simulink model "rlHouseHeatingSystem"  (R2023a)
settings: Solver=VariableStepAuto  StartTime=0.0  StopTime=inf  FixedStep=1  MaxStep=50  RelTol=1e-3  AbsTol=1e-3
InitFcn:
  | %   Simscape Demo "House Heating System"
  | % max_temp = 23;    % Maximum temperature
  | % min_temp = 18;     % Minimum temperature
  | % Walls
  | % House length = 30 m
  | lenHouse = 30;
  | % House width = 10 m
  | widHouse = 10;
  | % House height = 4 m
  | htHouse = 4;
  | wallArea = 2*lenHouse*htHouse + 2*widHouse*htHouse;
  | LWall = .2;
  | wallVolume = wallArea * LWall;
  | wallDensity = 1920;     % kg/m^3
  | wallMass = wallVolume * wallDensity;
  | c_wall = 835;           % J/kg/K
  | kWall = 0.038;  % Thermal conductivity [W/m/K]
  | % -------------------------------
  | % Windows
  | % Number of windows = 6
  | numWindows = 6;
  | % Height of windows = 1 m
  | htWindows = 1;
  | % Width of windows = 1 m
  | widWindows = 1;
  | windowArea = numWindows*htWindows*widWindows;
  | LWindow = .01;
  | windowVolume = windowArea * LWindow;
  | windowDensity = 2700;       % kg/m^3
  | windowMass = windowVolume * windowDensity;
  | c_window = 840;             % J/kg/K
  | kWindow = 0.78;             % Thermal conductivity [W/m/K]
  | % -------------------------------
  | % Roof
  | % Roof pitch = 40 deg
  | pitRoof = 40/180/pi;
  | roofArea =  2*(1/cos(pitRoof/2))*widHouse*lenHouse + tan(pitRoof)*widHouse;
  | LRoof = 0.2;
  | roofVolume = roofArea * LRoof;
  | roofDensity = 32;           % Glass fiber
  | roofMass = roofVolume * roofDensity;
  | kRoof = 0.038;              % Thermal conductivity [W/m/K]
  | c_roof = 835;               % J/kg/K
  | % -------------------------------
  | % Convective heat gransfer coefficients (W/M^2/K)
  | h_A_W = 24;         % Air-wall
  | h_W_Atm = 34;       % Wall-atmosphere
  | h_A_Wnd = 25;       % Air-window
  | h_Wnd_Atm = 32;     % Window-atmosphere
  | h_A_R = 12;         % Air-roof
  | h_R_Atm = 38;       % Roof-atmosphere
  | % -------------------------------
  | %Air
  | % Density of air at sea level = 1.2250 kg/m^3
  | densAir = 1.2250;
  | % Air mass inside the house
  | M_air = (lenHouse*widHouse*htHouse+tan(pitRoof)*widHouse*lenHouse)*densAir;
  | c_air = 1005.4;         % cp of air at 273 K [J/(kg*K]
  | % -------------------------------
  | % Heater
  | % The air exiting the heater has a constant temperature which is a heater
  | % property. THeater = 50 deg C
  | THeater = 50;
  | HeaterAirFlow = 1;  % Heater air flow rate [kg/s]
  | % -------------------------------
  | % Cost of electricity
  | % Assume the cost of electricity is $0.09 per kilowatt/hour
  | % Assume all electric energy is transformed to heat energy
  | % 1 kW-hr = 3.6e6 J
  | % cost = $0.09 per 3.6e6 J
  | cost = 0.09/3.6e6;
  | % -------------------------------
  | % Initial internal temperatures
  | TinIC = 20; % deg C
values from neighbouring files (symbols this model uses):
  comfortMax = 23    [1_initialhouseheatingmodel.m]
  comfortMin = 18    [1_initialhouseheatingmodel.m]
libraries: fl_lib x22, nesl_utility_internal x4, rllib x1
CloseFcn:
  | try,close(h1_ssc_house_heating_system),end
  | try,close(h2_ssc_house_heating_system),end
  | clear h1_ssc_house_heating_system h2_ssc_house_heating_system
  | 
  | clear simlog_ssc_house_heating_system
Description:
  | House Heating System
settings Model: ExtModeTrigMode=oneshot  Creator=The MathWorks, Inc.  LastModifiedBy=gcampa
settings SolverCC: AutoScaleAbsTol=off  AlgebraicLoopSolver=TrustRegion
settings DataIOCC: ExternalInput=[]  FinalStateName=Cost  InitialState=[]  SaveFormat=Array  SaveOutput=off  DSMLogging=off  SaveTime=off  SignalLoggingName=househeat_output
settings OptimizationCC: BlockReduction=off  BooleanDataType=off  ReuseModelBlockBuffer=off  ExpressionDepthLimit=2147483647  InitFltsAndDblsToZero=on  LifeSpan=inf  BufferReusableBoundary=off
settings DebuggingCC: SaveWithParameterizedLinksMsg=none  UnderspecifiedInitializationDetection=Classic  MergeDetectMultiDrivingBlocksExec=none  SignalResolutionControl=TryResolveAllWithWarning  MultiTaskDSMMsg=warning  MultiTaskCondExecSysMsg=none  IntegerOverflowMsg=none  FcnCallInpInsideContextMsg=warning  UnconnectedInputMsg=warning  UnconnectedOutputMsg=warning  UnconnectedLineMsg=warning  BusObjectLabelMismatch=none  AllowSymbolicDim=off  StateNameClashWarn=warning  PregeneratedLibrarySubsystemCodeDiagnostic=none  SFUnexpectedBacktrackingDiag=warning  SFNoUnconditionalDefaultTransitionDiag=warning  SFExecutionAtInitializationDiag=none  IntegerSaturationMsg=none  ArithmeticOperatorsInVariantConditions=warning
settings HardwareCC: ProdBitPerPointer=32  ProdBitPerSizeT=32  ProdBitPerPtrDiffT=32  ProdLargestAtomicFloat=None  ProdIntDivRoundTo=Undefined  ProdEndianess=Unspecified  ProdWordSize=32  ProdHWDeviceType=32-bit Generic  TargetUnknown=on
settings ModelReferenceCC: EnableRefExpFcnMdlSchedulingChecks=on  PropagateSignalLabelsOutOfModel=off
settings SFSimCC: SimUseLocalCustomCode=off  SimParseCustomCode=off  CustomCodeUndefinedFunction=UseInterfaceOnly
settings RTWCC: RTWUseLocalCustomCode=off  DLArmComputeVersion=19.05
settings CodeAppCC: StateflowObjectComments=on
settings GRTTargetCC: TargetFcnLib=ansi_tfl_tmw.mat  TargetLangStandard=C89/C90 (ANSI)  CombineOutputUpdateFcns=off  GRTInterface=on
settings ConfigComp: CovMetricSettings=dw  CovSaveCumulativeToWorkspaceVar=on  CovSaveSingleToWorkspaceVar=on  CovExternalEMLEnable=off  CovSFcnEnable=off
settings SimscapeCC: SimscapeLogName=simlog_ssc_house_heating_system  SimscapeLogDataHistory=25000

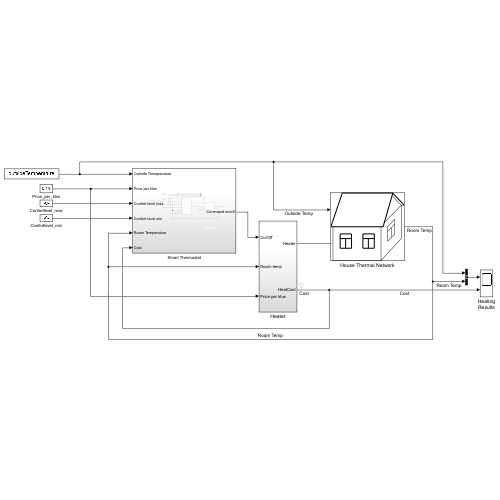
[thumbnail: Simulink's stored preview of the top-level diagram]
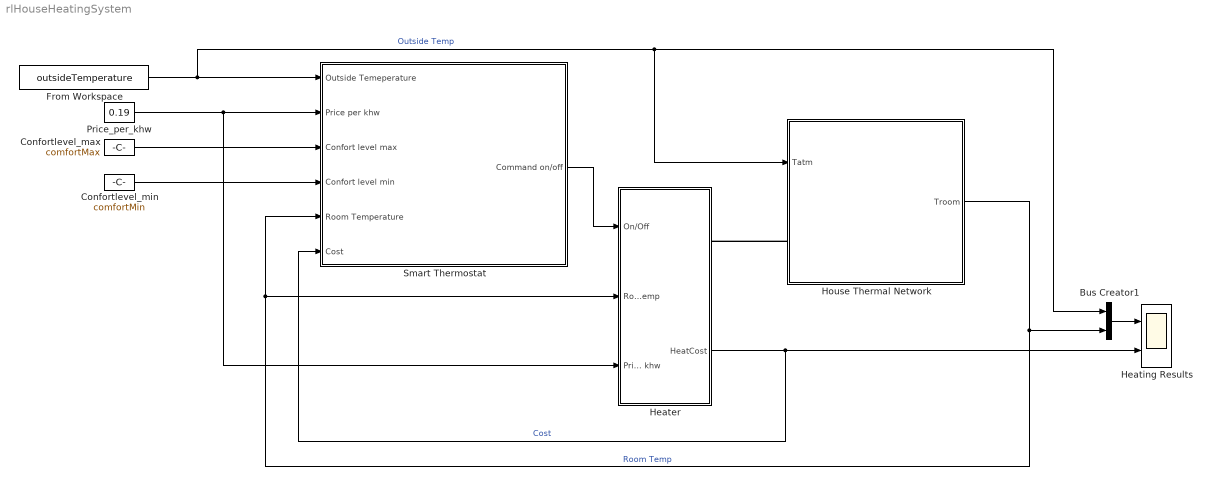
== system rlHouseHeatingSystem ==
  Bus Creator1 : BusCreator  Inputs=2
  Confortlevel_max : Constant  Value=comfortMax
  Confortlevel_min : Constant  Value=comfortMin
  From Workspace : FromWorkspace  VariableName=outsideTemperature
  Heater : Subsystem
      settings: PortSchema="{\"entries\":[{\"content\":{\"sides\":[{\"content\":{\"connectorIds\":[\"In1\",\"In2\",\"In3\"]},\"type\":\"ConnectorPlacement.EquallySpacedRectSide\",\"uuid\":\"6e4213b2-fad2-4bc5-9edd-55037a2291e4\"},{\"content\":{\"connectorIds\":[\"RConn1\",\"Out1\"],\"side\":\"RIGHT\"},\"type\":\"ConnectorPlacement.EquallySpacedRectSide\",\"uuid\":\"99418c11-ceb5-48dc-9314-931c2b0f004b\"},{\"content\":{\"connectorIds\":[],\"side\":\"TOP\"},\"type\":\"ConnectorPlacement.EquallySpacedRectSide\",\"uuid\":\"ba1c8d44-0580-4250-85f3-b0a12b6a254b\"}]},\"type\":\"ConnectorPlacement.EquallySpacedConnector\",\"uuid\":\"857183b6-2702-48a2-aa76-931984538a1b\"}],\"packageUris\":[\"http://schema.mathworks.com/mf0/Connector/R2020b\"],\"version\":\"1.0\"}"
  Heating Results : Scope  NumInputPorts=2
  House Thermal Network : Subsystem  Tag=PublishSubsystem
      mask Display:
      | plot([99.4454661849886;170.309218810871;170.309218810871;99.4454661849886;99.4454661849886], [212.827470386401;212.827470386401;127.790967235342;127.790967235342;212.827470386401])
      | plot([99.4454661849886;170.309218810871], [184.481969336048;184.481969336048])
      | plot([133.460067445412;133.460067445412], [184.481969336048;127.790967235342])
      | plot([241.172971436754;312.036724062636;312.036724062636;241.172971436754;241.172971436754], [212.827470386401;212.827470386401;127.790967235342;127.790967235342;212.827470386401])
      | plot([241.172971436754;312.036724062636], [184.481969336048;184.481969336048])
      | plot([275.187572697178;275.187572697178], [184.481969336048;127.790967235342])
      | plot([113.618216710165;42.7544640842825;368.727726163343;428.253278369084], [453.764229314402;255.34572196193;255.34572196193;453.764229314402])
      | plot([428.253278369084;499.117030994967], [453.764229314402;382.900476688519])
      | plot([113.618216710165;428.253278369084], [453.764229314402;453.764229314402])
      | plot([498.86507098563;499.368991004303], [382.900476688519;382.900476688519])
      | plot([482.109730364755;496.282480889931], [382.900476688519;382.900476688519])
      | plot([482.109730364755;374.396826373413], [382.900476688519;275.187572697178])
      | plot([482.109730364755;425.418728264049], [382.900476688519;439.591478789225])
      | plot([56.927214609459;56.927214609459;354.554975638166], [255.34572196193;56.927214609459;56.927214609459])
      | plot([354.554975638166;354.554975638166], [56.927214609459;255.34572196193])
      | plot([354.554975638166;482.109730364755;482.109730364755], [56.927214609459;184.481969336048;382.900476688519])
      | plot([397.073227213696;397.073227213696;439.591478789225;439.591478789225;397.073227213696], [170.309218810871;255.34572196193;297.86397353746;209.992920281366;170.309218810871])
      | plot([397.073227213696;439.591478789225], [227.000220911577;269.518472487107])
      | plot([419.749628053978;419.749628053978], [246.842071646824;192.985619651154])
      | %patch([0;553.20969549939;553.20969549939;0;0;0.472425017505884;0.47242501750577;552.737270481884;552.737270481885;0.472425017505884;0], [496.518693398684;496.518693398684;0;0;496.518693398684;496.046268381178;0.472425017505884;0.472425017505884;496.046268381178;496.046268381178;496.518693398684], [1;1;1])
  Price_per_khw : Constant  Value=0.19
  Smart Thermostat : Subsystem
  wires:
  House Thermal Network/1(Troom) -> Smart Thermostat/5(Room Temperature), Heater/2(Room temp), Bus Creator1/2  "Room Temp"
  From Workspace/1 -> House Thermal Network/1(Tatm), Bus Creator1/1, Smart Thermostat/1(Outside Temeperature)  "Outside Temp"
  Bus Creator1/1 -> Heating Results/1
  Heater/1(HeatCost) -> Smart Thermostat/6(Cost), Heating Results/2  "Cost"
  Price_per_khw/1 -> Heater/3(Price per khw), Smart Thermostat/2(Price per khw)
  Confortlevel_max/1 -> Smart Thermostat/3(Confort level max)
  Confortlevel_min/1 -> Smart Thermostat/4(Confort level min)
  Smart Thermostat/1(Command on/off) -> Heater/1(On/Off)
  connections:
  House Thermal Network/LConn1 -- Heater/RConn1

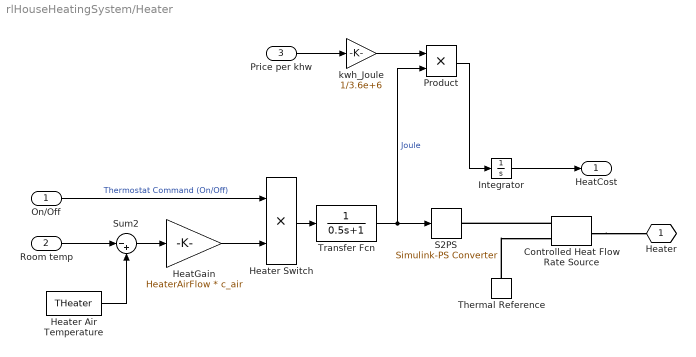
== system rlHouseHeatingSystem/Heater ==
  On/Off : Inport
  Room temp : Inport  Port=2
  Price per khw : Inport  Port=3
  Controlled Heat Flow Rate Source : fl_lib/Thermal/Thermal Sources/Controlled Heat Flow Rate Source
  HeatGain : Gain  Gain=HeaterAirFlow * c_air
  Heater Air Temperature : Constant  Value=THeater
  Heater Switch : Product  RndMeth=Zero
  Integrator : Integrator
  Product : Product
  S2PS : nesl_utility_internal/Simulink-PS Converter  PhysicalDomain=network_engine_domain  SubClassName=ps_input  LeftPortType=input  RightPortType=output  PseudoPeriodic=off  Frequencies=[]  NoiseDistribution=none  NoiseParameters=[]  Unit=1  AffineConversion=off  FilteringAndDerivatives=zero  SimscapeFilterOrder=1  InputFilterTimeConstant=.001  UdotUserProvided=0
  Sum2 : Sum  Inputs=|-+
  Thermal Reference : fl_lib/Thermal/Thermal Elements/Thermal Reference
  Transfer Fcn : TransferFcn  Denominator=[0.5 1]
  kwh_Joule : Gain  Gain=1/3.6e+6
  Heater : PMIOPort  Tag=PMCPort  Side=Right
  HeatCost : Outport  VectorParamsAs1DForOutWhenUnconnected=off
  wires:
  Heater Air Temperature/1 -> Sum2/2
  Room temp/1 -> Sum2/1
  Sum2/1 -> HeatGain/1
  On/Off/1 -> Heater Switch/1  "Thermostat Command (On/Off)"
  HeatGain/1 -> Heater Switch/2
  Heater Switch/1 -> Transfer Fcn/1
  Integrator/1 -> HeatCost/1
  Transfer Fcn/1 -> S2PS/1, Product/2  "Joule"
  Price per khw/1 -> kwh_Joule/1
  kwh_Joule/1 -> Product/1
  Product/1 -> Integrator/1
  connections:
  Controlled Heat Flow Rate Source/RConn1 -- S2PS/RConn1
  Thermal Reference/LConn1 -- Controlled Heat Flow Rate Source/RConn2
  Controlled Heat Flow Rate Source/LConn1 -- Heater/RConn1

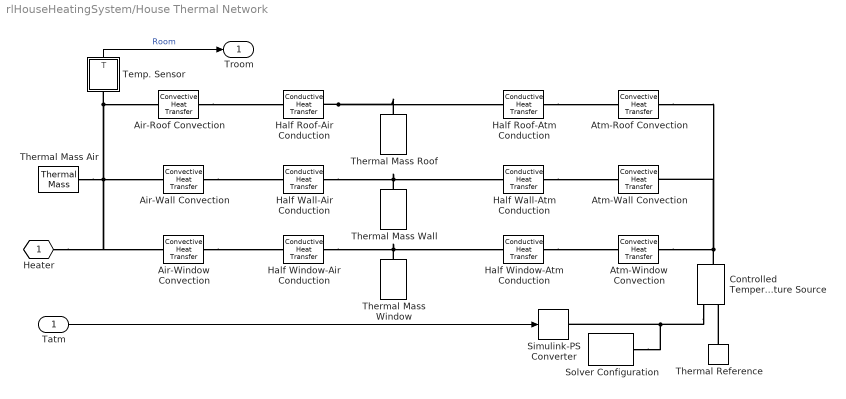
== system rlHouseHeatingSystem/House Thermal Network ==
  Tatm : Inport
  Air-Roof Convection : fl_lib/Thermal/Thermal Elements/Convective Heat Transfer  thermal_type=foundation.enum.constant_variable.constant  area=roofArea m^2  heat_tr_coeff=h_A_R W/m^2/K  min_heat_tr_coeff=1e-3 W/(K*m^2)  T_specify=off  T_priority=High  T=0 K  T_nominal_specify=off  T_nominal_unit=K  T_nominal_value=1  Q_specify=off  Q_priority=High  Q=0 J/s  Q_nominal_specify=off  Q_nominal_unit=W  Q_nominal_value=1
  Air-Wall Convection : fl_lib/Thermal/Thermal Elements/Convective Heat Transfer  thermal_type=foundation.enum.constant_variable.constant  area=wallArea m^2  heat_tr_coeff=h_A_W W/m^2/K  min_heat_tr_coeff=1e-3 W/(K*m^2)  T_specify=off  T_priority=High  T=0 K  T_nominal_specify=off  T_nominal_unit=K  T_nominal_value=1  Q_specify=off  Q_priority=High  Q=0 J/s  Q_nominal_specify=off  Q_nominal_unit=W  Q_nominal_value=1
  Air-Window Convection : fl_lib/Thermal/Thermal Elements/Convective Heat Transfer  thermal_type=foundation.enum.constant_variable.constant  area=windowArea m^2  heat_tr_coeff=h_A_Wnd W/m^2/K  min_heat_tr_coeff=1e-3 W/(K*m^2)  T_specify=off  T_priority=High  T=0 K  T_nominal_specify=off  T_nominal_unit=K  T_nominal_value=1  Q_specify=off  Q_priority=High  Q=0 J/s  Q_nominal_specify=off  Q_nominal_unit=W  Q_nominal_value=1
  Atm-Roof Convection : fl_lib/Thermal/Thermal Elements/Convective Heat Transfer  thermal_type=foundation.enum.constant_variable.constant  area=roofArea m^2  heat_tr_coeff=h_R_Atm W/m^2/K  min_heat_tr_coeff=1e-3 W/(K*m^2)  T_specify=off  T_priority=High  T=0 K  T_nominal_specify=off  T_nominal_unit=K  T_nominal_value=1  Q_specify=off  Q_priority=High  Q=0 J/s  Q_nominal_specify=off  Q_nominal_unit=W  Q_nominal_value=1
  Atm-Wall Convection : fl_lib/Thermal/Thermal Elements/Convective Heat Transfer  thermal_type=foundation.enum.constant_variable.constant  area=wallArea m^2  heat_tr_coeff=h_W_Atm W/m^2/K  min_heat_tr_coeff=1e-3 W/(K*m^2)  T_specify=off  T_priority=High  T=0 K  T_nominal_specify=off  T_nominal_unit=K  T_nominal_value=1  Q_specify=off  Q_priority=High  Q=0 J/s  Q_nominal_specify=off  Q_nominal_unit=W  Q_nominal_value=1
  Atm-Window Convection : fl_lib/Thermal/Thermal Elements/Convective Heat Transfer  thermal_type=foundation.enum.constant_variable.constant  area=windowArea m^2  heat_tr_coeff=h_Wnd_Atm W/m^2/K  min_heat_tr_coeff=1e-3 W/(K*m^2)  T_specify=off  T_priority=High  T=0 K  T_nominal_specify=off  T_nominal_unit=K  T_nominal_value=1  Q_specify=off  Q_priority=High  Q=0 J/s  Q_nominal_specify=off  Q_nominal_unit=W  Q_nominal_value=1
  Controlled Temperature Source : fl_lib/Thermal/Thermal Sources/Controlled Temperature Source
  Half Roof-Air Conduction : fl_lib/Thermal/Thermal Elements/Conductive Heat Transfer  thermal_type=foundation.enum.ConstantVariableTabulated.Constant  wall_geometry=foundation.enum.ConductionWallGeometry.Planar  area=roofArea m^2  thickness=LRoof/2 m  d_in=0.05 m  d_out=0.1 m  L=1 m  th_cond_min=10 W/(K*m)  th_cond=kRoof W/m/K  th_cond_TLU=[413, 401, 392, 383, 371, 357, 342] W/(K*m)  temp_TLU=[200, 273, 400, 600, 800, 1000, 1200] K  T_specify=off  T_priority=High  T=0 K  T_nominal_specify=off  T_nominal_unit=K  T_nominal_value=1  Q_specify=off  Q_priority=High  Q=0 J/s  Q_nominal_specify=off  Q_nominal_unit=W  Q_nominal_value=1
  Half Roof-Atm Conduction : fl_lib/Thermal/Thermal Elements/Conductive Heat Transfer  thermal_type=foundation.enum.ConstantVariableTabulated.Constant  wall_geometry=foundation.enum.ConductionWallGeometry.Planar  area=roofArea m^2  thickness=LRoof/2 m  d_in=0.05 m  d_out=0.1 m  L=1 m  th_cond_min=10 W/(K*m)  th_cond=kRoof W/m/K  th_cond_TLU=[413, 401, 392, 383, 371, 357, 342] W/(K*m)  temp_TLU=[200, 273, 400, 600, 800, 1000, 1200] K  T_specify=off  T_priority=High  T=0 K  T_nominal_specify=off  T_nominal_unit=K  T_nominal_value=1  Q_specify=off  Q_priority=High  Q=0 J/s  Q_nominal_specify=off  Q_nominal_unit=W  Q_nominal_value=1
  Half Wall-Air Conduction : fl_lib/Thermal/Thermal Elements/Conductive Heat Transfer  thermal_type=foundation.enum.ConstantVariableTabulated.Constant  wall_geometry=foundation.enum.ConductionWallGeometry.Planar  area=wallArea m^2  thickness=LWall/2 m  d_in=0.05 m  d_out=0.1 m  L=1 m  th_cond_min=10 W/(K*m)  th_cond=kWall W/m/K  th_cond_TLU=[413, 401, 392, 383, 371, 357, 342] W/(K*m)  temp_TLU=[200, 273, 400, 600, 800, 1000, 1200] K  T_specify=off  T_priority=High  T=0 K  T_nominal_specify=off  T_nominal_unit=K  T_nominal_value=1  Q_specify=off  Q_priority=High  Q=0 J/s  Q_nominal_specify=off  Q_nominal_unit=W  Q_nominal_value=1
  Half Wall-Atm Conduction : fl_lib/Thermal/Thermal Elements/Conductive Heat Transfer  thermal_type=foundation.enum.ConstantVariableTabulated.Constant  wall_geometry=foundation.enum.ConductionWallGeometry.Planar  area=wallArea m^2  thickness=LWall/2 m  d_in=0.05 m  d_out=0.1 m  L=1 m  th_cond_min=10 W/(K*m)  th_cond=kWall W/m/K  th_cond_TLU=[413, 401, 392, 383, 371, 357, 342] W/(K*m)  temp_TLU=[200, 273, 400, 600, 800, 1000, 1200] K  T_specify=off  T_priority=High  T=0 K  T_nominal_specify=off  T_nominal_unit=K  T_nominal_value=1  Q_specify=off  Q_priority=High  Q=0 J/s  Q_nominal_specify=off  Q_nominal_unit=W  Q_nominal_value=1
  Half Window-Air Conduction : fl_lib/Thermal/Thermal Elements/Conductive Heat Transfer  thermal_type=foundation.enum.ConstantVariableTabulated.Constant  wall_geometry=foundation.enum.ConductionWallGeometry.Planar  area=windowArea m^2  thickness=LWindow/2 m  d_in=0.05 m  d_out=0.1 m  L=1 m  th_cond_min=10 W/(K*m)  th_cond=kWindow W/m/K  th_cond_TLU=[413, 401, 392, 383, 371, 357, 342] W/(K*m)  temp_TLU=[200, 273, 400, 600, 800, 1000, 1200] K  T_specify=off  T_priority=High  T=0 K  T_nominal_specify=off  T_nominal_unit=K  T_nominal_value=1  Q_specify=off  Q_priority=High  Q=0 J/s  Q_nominal_specify=off  Q_nominal_unit=W  Q_nominal_value=1
  Half Window-Atm Conduction : fl_lib/Thermal/Thermal Elements/Conductive Heat Transfer  thermal_type=foundation.enum.ConstantVariableTabulated.Constant  wall_geometry=foundation.enum.ConductionWallGeometry.Planar  area=windowArea m^2  thickness=LWindow/2 m  d_in=0.05 m  d_out=0.1 m  L=1 m  th_cond_min=10 W/(K*m)  th_cond=kWindow W/m/K  th_cond_TLU=[413, 401, 392, 383, 371, 357, 342] W/(K*m)  temp_TLU=[200, 273, 400, 600, 800, 1000, 1200] K  T_specify=off  T_priority=High  T=0 K  T_nominal_specify=off  T_nominal_unit=K  T_nominal_value=1  Q_specify=off  Q_priority=High  Q=0 J/s  Q_nominal_specify=off  Q_nominal_unit=W  Q_nominal_value=1
  Simulink-PS Converter : nesl_utility_internal/Simulink-PS Converter  PhysicalDomain=network_engine_domain  SubClassName=ps_input  LeftPortType=input  RightPortType=output  PseudoPeriodic=off  Frequencies=[]  NoiseDistribution=none  NoiseParameters=[]  Unit=degC  AffineConversion=on  FilteringAndDerivatives=zero  SimscapeFilterOrder=1  InputFilterTimeConstant=.001  UdotUserProvided=0
  Solver Configuration : nesl_utility_internal/Solver Configuration  PhysicalDomain=network_engine_domain  SubClassName=solver  LeftPortType=input  RightPortType=generic  Tones=[]  Harmonics=[]  SimulateNoise=off  Profile=off  UseLocalSampling=off  EnableSwitchedLinearOptims=on  FrequencyDomain=off  UseCCode=off  RelTol=0.001  AbsTol=1e-06  MinStep=1e-09  ToWorkspace=off  RevertToSquareIcSolve=off  NumHomotopyIterations=100  PhasorMode=off  PhasorModeNumHarmonics=1  ConsistencySolver=NEWTON_FTOL  IndexReductionMethod=DerivativeReplacement  DoDC=off  ResidualTolerance=1e-9  ConsistencyTolSource=GLOBAL  ConsistencyAbsTol=0.001  ConsistencyRelTol=0.001  ConsistencyTolFactor=0.001  UseLocalSolver=off  LocalSolverChoice=NE_BACKWARD_EULER_ADVANCER  ResolveIndetEquations=on  FunctionEvalNumThread=1  LocalSolverSampleTime=.001  DoFixedCost=off  MaxNonlinIter=3  MaxModeIter=2  ComputeImpulses=off  ImpulseIterations=2  LinearAlgebra=auto  LinearAlgebraNumThread=0  EquationFormulation=NE_TIME_EF  DelaysMemoryBudget=1024  AutomaticFiltering=on  FilteringTimeConstant=0.001  PartitionStorageMethod=AS_NEEDED  PartitionMemoryBudget=1024  PartitionMethod=FAST
  Temp. Sensor : Subsystem
  Thermal Mass Air : fl_lib/Thermal/Thermal Elements/Thermal Mass  mass_type=foundation.enum.constant_variable.constant  mass=M_air kg  sp_heat=c_air J/kg/K  mass_min=1e-6 kg  num_ports=foundation.enum.numPorts2.one  m_specify=off  m_priority=High  m=1 kg  m_nominal_specify=off  m_nominal_unit=kg  m_nominal_value=1  T_specify=on  T_priority=High  T=TinIC degC  T_nominal_specify=off  T_nominal_unit=K  T_nominal_value=1  Q_specify=off  Q_priority=None  Q=0 W  Q_nominal_specify=off  Q_nominal_unit=W  Q_nominal_value=1
  Thermal Mass Roof : fl_lib/Thermal/Thermal Elements/Thermal Mass  mass_type=foundation.enum.constant_variable.constant  mass=roofMass kg  sp_heat=c_roof J/kg/K  mass_min=1e-6 kg  num_ports=foundation.enum.numPorts2.one  m_specify=off  m_priority=High  m=1 kg  m_nominal_specify=off  m_nominal_unit=kg  m_nominal_value=1  T_specify=on  T_priority=High  T=TinIC degC  T_nominal_specify=off  T_nominal_unit=K  T_nominal_value=1  Q_specify=off  Q_priority=None  Q=0 W  Q_nominal_specify=off  Q_nominal_unit=W  Q_nominal_value=1
  Thermal Mass Wall : fl_lib/Thermal/Thermal Elements/Thermal Mass  mass_type=foundation.enum.constant_variable.constant  mass=wallMass kg  sp_heat=c_wall J/kg/K  mass_min=1e-6 kg  num_ports=foundation.enum.numPorts2.one  m_specify=off  m_priority=High  m=1 kg  m_nominal_specify=off  m_nominal_unit=kg  m_nominal_value=1  T_specify=on  T_priority=High  T=TinIC degC  T_nominal_specify=off  T_nominal_unit=K  T_nominal_value=1  Q_specify=off  Q_priority=None  Q=0 W  Q_nominal_specify=off  Q_nominal_unit=W  Q_nominal_value=1
  Thermal Mass Window : fl_lib/Thermal/Thermal Elements/Thermal Mass  mass_type=foundation.enum.constant_variable.constant  mass=windowMass kg  sp_heat=c_window J/kg/K  mass_min=1e-6 kg  num_ports=foundation.enum.numPorts2.one  m_specify=off  m_priority=High  m=1 kg  m_nominal_specify=off  m_nominal_unit=kg  m_nominal_value=1  T_specify=on  T_priority=High  T=TinIC degC  T_nominal_specify=off  T_nominal_unit=K  T_nominal_value=1  Q_specify=off  Q_priority=None  Q=0 W  Q_nominal_specify=off  Q_nominal_unit=W  Q_nominal_value=1
  Thermal Reference : fl_lib/Thermal/Thermal Elements/Thermal Reference
  Heater : PMIOPort  Tag=PMCPort  Side=Left
  Troom : Outport  InitialOutput=0  VectorParamsAs1DForOutWhenUnconnected=off
  wires:
  Tatm/1 -> Simulink-PS Converter/1
  Temp. Sensor/1(T) -> Troom/1  "Room"
  connections:
  Thermal Reference/LConn1 -- Controlled Temperature Source/RConn2
  Solver Configuration/RConn1 -- Controlled Temperature Source/RConn1 -- Simulink-PS Converter/RConn1
  Heater/RConn1 -- Air-Window Convection/LConn1 -- Thermal Mass Air/LConn1 -- Air-Wall Convection/LConn1 -- Air-Roof Convection/LConn1 -- Temp. Sensor/LConn1
  Air-Wall Convection/RConn1 -- Half Wall-Air Conduction/LConn1
  Half Wall-Air Conduction/RConn1 -- Thermal Mass Wall/LConn1 -- Half Wall-Atm Conduction/LConn1
  Half Wall-Atm Conduction/RConn1 -- Atm-Wall Convection/LConn1
  Air-Window Convection/RConn1 -- Half Window-Air Conduction/LConn1
  Half Window-Air Conduction/RConn1 -- Thermal Mass Window/LConn1 -- Half Window-Atm Conduction/LConn1
  Half Window-Atm Conduction/RConn1 -- Atm-Window Convection/LConn1
  Air-Roof Convection/RConn1 -- Half Roof-Air Conduction/LConn1
  Half Roof-Air Conduction/RConn1 -- Half Roof-Atm Conduction/LConn1 -- Thermal Mass Roof/LConn1
  Half Roof-Atm Conduction/RConn1 -- Atm-Roof Convection/LConn1
  Atm-Window Convection/RConn1 -- Controlled Temperature Source/LConn1 -- Atm-Roof Convection/RConn1 -- Atm-Wall Convection/RConn1

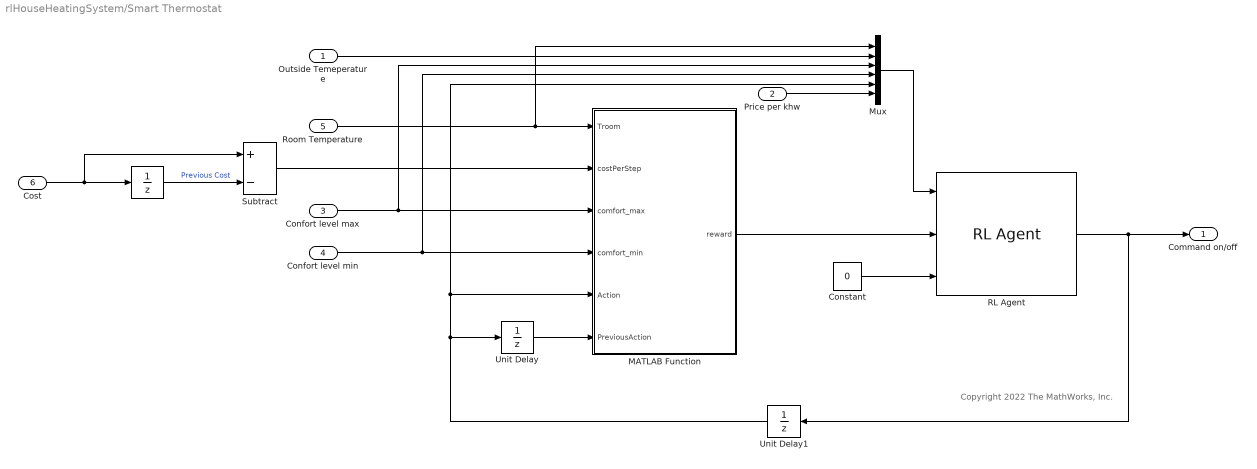
== system rlHouseHeatingSystem/Smart Thermostat ==
  note: Copyright 2022 The MathWorks, Inc.
  Outside Temeperature : Inport
  Price per khw : Inport  Port=2
  Confort level max : Inport  Port=3
  Confort level min : Inport  Port=4
  Room Temperature : Inport  Port=5
  Cost : Inport  Port=6
  " " : UnitDelay  SampleTime=-1  HasFrameUpgradeWarning=on
  Constant : Constant  Value=0
  MATLAB Function : MATLAB Function  TreatAsAtomicUnit=on
  Mux : Mux  Inputs=6
  RL Agent : rllib/RL Agent  Agent=agent  ExternalActionAsInput=off  ProvideLastAction=off  ProvideCumRwd=off  TreatAsDirectFeedthrough=on  UseStrictObservationDataTypes=off
  Subtract : Sum  Inputs=+-
  Unit Delay : UnitDelay  SampleTime=-1  HasFrameUpgradeWarning=on
  Unit Delay1 : UnitDelay  SampleTime=-1  HasFrameUpgradeWarning=on
  Command on/off : Outport
  wires:
  RL Agent/1 -> Command on/off/1, Unit Delay1/1
  Subtract/1 -> MATLAB Function/2(costPerStep)
  Unit Delay1/1 -> Mux/5, MATLAB Function/5(Action), Unit Delay/1
  Unit Delay/1 -> MATLAB Function/6(PreviousAction)
  Constant/1 -> RL Agent/3
  Outside Temeperature/1 -> Mux/2
  Cost/1 -> Subtract/1, " "/1
  Confort level min/1 -> Mux/4, MATLAB Function/4(comfort_min)
  Confort level max/1 -> Mux/3, MATLAB Function/3(comfort_max)
  MATLAB Function/1(reward) -> RL Agent/2
  Mux/1 -> RL Agent/1
  " "/1 -> Subtract/2  "Previous Cost"
  Room Temperature/1 -> Mux/1, MATLAB Function/1(Troom)
  Price per khw/1 -> Mux/6

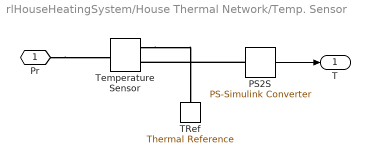
== system rlHouseHeatingSystem/House Thermal Network/Temp. Sensor ==
  PS2S : nesl_utility_internal/PS-Simulink Converter  PhysicalDomain=network_engine_domain  SubClassName=ps_output  LeftPortType=input  RightPortType=output  PseudoPeriodic=off  Frequencies=[]  VectorFormat=1-D array  Unit=degC  AffineConversion=on
  TRef : fl_lib/Thermal/Thermal Elements/Thermal Reference
  Temperature Sensor : fl_lib/Thermal/Thermal Sensors/Temperature Sensor
  Pr : PMIOPort  Side=Left
  T : Outport  VectorParamsAs1DForOutWhenUnconnected=off
  wires:
  PS2S/1 -> T/1
  connections:
  Temperature Sensor/RConn1 -- TRef/LConn1
  PS2S/LConn1 -- Temperature Sensor/RConn2
  Pr/RConn1 -- Temperature Sensor/LConn1

== matlab function rlHouseHeatingSystem/Smart Thermostat/MATLAB Function ==
  data: Troom input; costPerStep input; reward output; comfort_max input; comfort_min input; Action input; PreviousAction input
function reward = rewardFcn(Troom, costPerStep, comfort_max, comfort_min, Action, PreviousAction)

% energy cost
energyReward  = -costPerStep;

% comfort level reward
if (Troom >= comfort_min) && (Troom <=comfort_max)
    comfortReward = 0.1;
elseif Troom < comfort_min    
    comfortReward = -0.1*abs(Troom - comfort_min);
elseif  Troom > comfort_max    
    comfortReward = -0.1*abs(Troom - comfort_max);
else 
    comfortReward = 0;
end

% switch penalty
if PreviousAction ~= Action
    switchPenalty = -0.01;
else
    switchPenalty = 0;
end

reward = energyReward + comfortReward + switchPenalty;
